simulink model "demoRPiSerialFrame"  (R2016a)
settings: Solver=FixedStepAuto  SolverMode=SingleTasking  StartTime=0.0  StopTime=inf  FixedStep=0.1  RelTol=1e-3
libraries: simulink x3, RPi x2
settings Model: SimulationMode=external  Creator=user  LastModifiedBy=user
settings SolverCC: PositivePriorityOrder=on
settings OptimizationCC: OptimizeModelRefInitCode=on  LifeSpan=1  MaxStackSize=64
settings HardwareCC: ProdBitPerPointer=32  ProdLargestAtomicInteger=Long  ProdLargestAtomicFloat=Double  ProdWordSize=32  ProdHWDeviceType=ARM Compatible->ARM Cortex
settings RTWCC: SystemTargetFile=ert.tlc  HardwareBoard=Raspberry Pi  TemplateMakefile=ert_default_tmf  GenerateReport=on  Toolchain=GNU GCC Raspberry Pi  IncludeHyperlinkInReport=on  LaunchReport=on  TargetLang=C++  GenerateTraceInfo=on  GenerateTraceReport=on  GenerateTraceReportSl=on  GenerateTraceReportSf=on  GenerateTraceReportEml=on
settings CodeAppCC: ForceParamTrailComments=on  IgnoreCustomStorageClasses=off  OperatorAnnotations=on  SimulinkDataObjDesc=on  SFDataObjDesc=on  MATLABFcnDesc=on  InsertBlockDesc=on  MATLABSourceComments=on
settings ERTTargetCC: SupportVariableSizeSignals=on

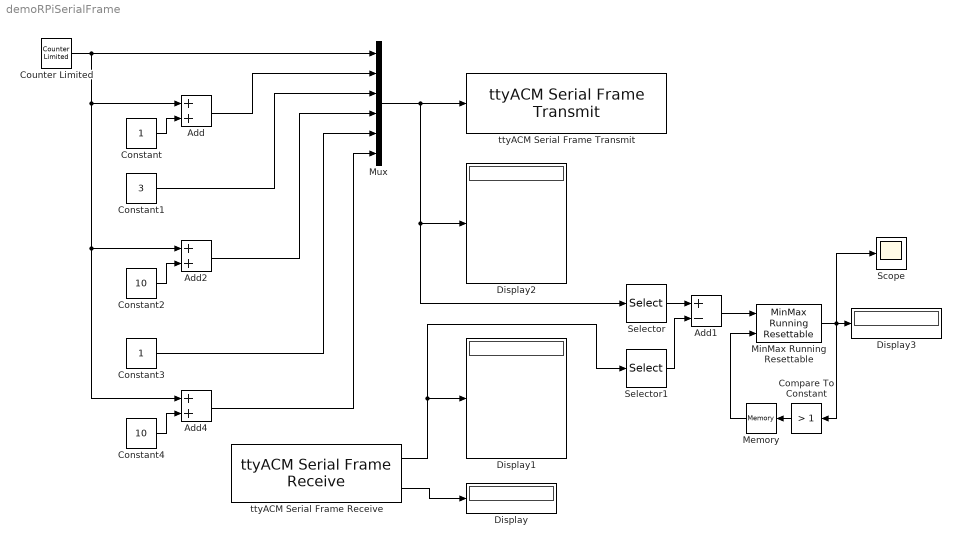
== system demoRPiSerialFrame ==
  Add : Sum
  Add1 : Sum  Inputs=+-
  Add2 : Sum
  Add4 : Sum
  Compare To Constant : simulink/Logic and Bit Operations/Compare To Constant  relop=>  const=1  OutDataTypeStr=boolean
  Constant : Constant  OutDataTypeStr=uint8
  Constant1 : Constant  Value=3  OutDataTypeStr=uint8
  Constant2 : Constant  Value=10  OutDataTypeStr=uint8
  Constant3 : Constant  OutDataTypeStr=uint8
  Constant4 : Constant  Value=10  OutDataTypeStr=uint8
  Counter Limited : simulink/Sources/Counter Limited  uplimit=200  tsamp=-1
  Display{,1..3} (4 alike) : Display
  Memory : Memory
  MinMax Running Resettable : simulink/Math Operations/MinMax Running Resettable  Function=max  vinit=0.0
  Mux : Mux  Inputs=6
  Scope : Scope
  Selector : Selector  InputPortWidth=6  IndexOptions=Index vector (dialog)  Indices=[1]  OutputSizes=1
  Selector1 : Selector  InputPortWidth=6  IndexOptions=Index vector (dialog)  Indices=[1]  OutputSizes=1
  ttyACM Serial Frame Receive : RPi/ttyACM Serial Frame Receive  portID=0  SOFbyte=254  EOFbyte=255  msgLen=6  SimulateUsing=Code generation
  ttyACM Serial Frame Transmit : RPi/ttyACM Serial Frame Transmit  portID=0  SOFbyte=254  EOFbyte=255  SimulateUsing=Code generation
  wires:
  Constant/1 -> Add/2
  Constant2/1 -> Add2/2
  Add/1 -> Mux/2
  Constant1/1 -> Mux/3
  Add2/1 -> Mux/4
  Mux/1 -> Selector/1, Display2/1, ttyACM Serial Frame Transmit/1
  ttyACM Serial Frame Receive/2 -> Display/1
  ttyACM Serial Frame Receive/1 -> Selector1/1, Display1/1
  Counter Limited/1 -> Mux/1, Add4/1, Add2/1, Add/1
  Constant4/1 -> Add4/2
  Constant3/1 -> Mux/5
  Add4/1 -> Mux/6
  Selector/1 -> Add1/1
  Selector1/1 -> Add1/2
  Add1/1 -> MinMax Running Resettable/1
  MinMax Running Resettable/1 -> Compare To Constant/1, Scope/1, Display3/1
  Memory/1 -> MinMax Running Resettable/2
  Compare To Constant/1 -> Memory/1
